simulink model "ammclib_gflib_trigonometric_s32k14x"  (Simulink 9.0)
settings: Solver=FixedStepDiscrete  StartTime=0.0  StopTime=5  FixedStep=0.001  RelTol=1e-3  EnableMultiTasking=on
InitFcn:
  | mbd_s32k_consistency_checks(bdroot(gcs));
undefined symbols (not defined in the file or in its folder): LQFP
libraries: ammclib_bam_s32k14x x70, mbd_s32k1xx_ec_toolbox x2, simulink x1
Description:
  | This model tests the AMMCLIB GFLIB TRIGONOMETRIC blocks
  | 
  | Validation:
  | - Run the model in Simulation and check the results
  | - Open Freemaster (ammclib_gflib_trigonometric_s32k14x.pmp) and compare the HW results against the Simulated ones
CloseFcn:
  | clear all;
settings Model: Creator=NXP MBDT Team  LastModifiedBy=nxf35172
settings DataIOCC: ExternalInput=off  InitialState=off  LimitDataPoints=on  SaveOutput=off  SignalLogging=off  SaveTime=off
settings OptimizationCC: DefaultParameterBehavior=Inlined  LifeSpan=1
settings DebuggingCC: SolverPrmCheckMsg=warning  InheritedTsInSrcMsg=none  SingleTaskRateTransMsg=error  IntegerOverflowMsg=none  ParameterPrecisionLossMsg=none  UnconnectedInputMsg=error  UnconnectedOutputMsg=error  UnconnectedLineMsg=error  AllowSymbolicDim=off  UnknownTsInhSupMsg=error  StateNameClashWarn=warning
settings HardwareCC: ProdLargestAtomicInteger=Long  ProdLargestAtomicFloat=Double  ProdEndianess=LittleEndian  ProdHWDeviceType=ARM Compatible->ARM Cortex
settings SFSimCC: MATLABDynamicMemAlloc=off
settings RTWCC: SystemTargetFile=mbd_s32k.tlc  MakeCommand=mbd_s32k_make_rtw COPY_MDLREF_INCLUDES=0  TemplateMakefile=mbd_s32k.tmf  Description=Model Based Design Toolbox S32K14x Code Generation Target
settings CodeAppCC: IgnoreCustomStorageClasses=off
settings STFCustomTargetCC: CombineOutputUpdateFcns=on  ERTCustomFileBanners=on  SupportContinuousTime=off  SupportNonInlinedSFcns=off  RemoveResetFunc=on  MATLABClassNameForMDSCustomization=Simulink.SoftwareTarget.ERTCustomization  GRTInterface=off  SystemTargetFile=mbd_s32k14.tlc
settings ERTTargetCC: MultiwordLength=2048  ParMdlRefBuildCompliant=off  CompOptLevelCompliant=off  ConcurrentExecutionCompliant=off  ModelStepFunctionPrototypeControlCompliant=off  CPPClassGenCompliant=off  UseToolchainInfoCompliant=off  InlinedParameterPlacement=NonHierarchical  ERTCustomFileTemplate=example_file_process.tlc  ConvertIfToSwitch=off  SuppressUnreachableDefaultCases=off

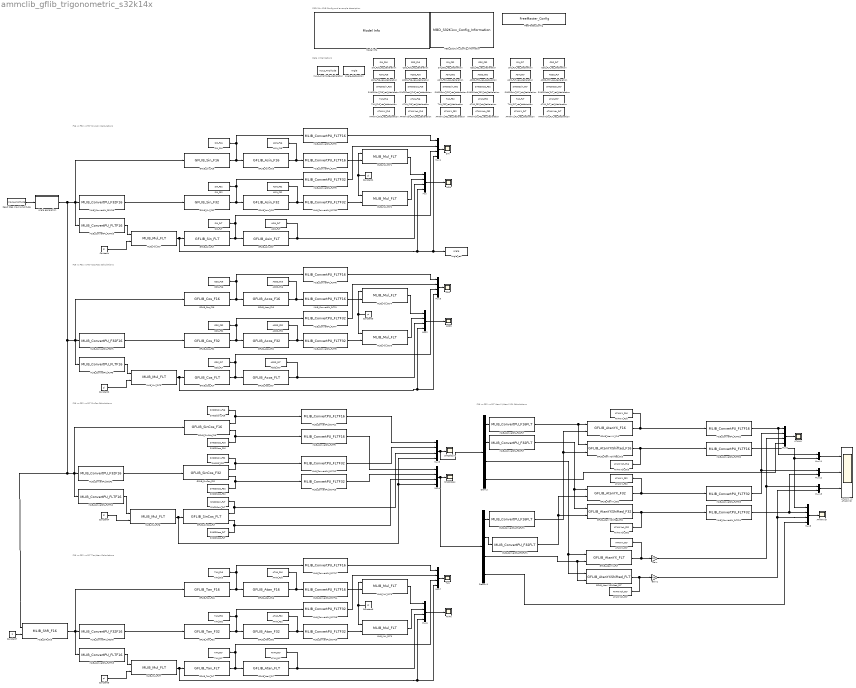
== system ammclib_gflib_trigonometric_s32k14x ==
  note: S32K14x EVB Config and example description
  note: Data Initializations
  note: F16 vs F32 vs FLT Sin/Asin Calculations
  note: F16 vs F32 vs FLT Cos/Acos Calculations
  note: F16 vs F32 vs FLT SinCos Calculations
  note: F16 vs F32 vs FLT Tan/Atan Calculations
  note: F16 vs F32 vs FLT AtanYX/AtanYXSh Calculations
  ACOS : Scope
  ACOS_F16 : DataStoreWrite  DataStoreName=ACOS_F16
  ACOS_F16_res_declaration : DataStoreMemory  Priority=2  DataStoreName=ACOS_F16  ReadBeforeWriteMsg=warning  WriteAfterWriteMsg=warning  WriteAfterReadMsg=warning  ShowAdditionalParam=off  OutDataTypeStr=int16
  ACOS_F32 : DataStoreWrite  DataStoreName=ACOS_F32
  ACOS_F32_res_declaration : DataStoreMemory  Priority=2  DataStoreName=ACOS_F32  ReadBeforeWriteMsg=warning  WriteAfterWriteMsg=warning  WriteAfterReadMsg=warning  ShowAdditionalParam=off  OutDataTypeStr=int32
  ACOS_FLT : DataStoreWrite  DataStoreName=ACOS_FLT
  ACOS_FLT_res_declaration : DataStoreMemory  Priority=2  DataStoreName=ACOS_FLT  ReadBeforeWriteMsg=warning  WriteAfterWriteMsg=warning  WriteAfterReadMsg=warning  ShowAdditionalParam=off  OutDataTypeStr=single
  ASIN : Scope
  ASIN_F16 : DataStoreWrite  DataStoreName=ASIN_F16
  ASIN_F16_res_declaration : DataStoreMemory  Priority=2  DataStoreName=ASIN_F16  ReadBeforeWriteMsg=warning  WriteAfterWriteMsg=warning  WriteAfterReadMsg=warning  ShowAdditionalParam=off  OutDataTypeStr=int16
  ASIN_F32 : DataStoreWrite  DataStoreName=ASIN_F32
  ASIN_F32_res_declaration : DataStoreMemory  Priority=2  DataStoreName=ASIN_F32  ReadBeforeWriteMsg=warning  WriteAfterWriteMsg=warning  WriteAfterReadMsg=warning  ShowAdditionalParam=off  OutDataTypeStr=int32
  ASIN_FLT : DataStoreWrite  DataStoreName=ASIN_FLT
  ASIN_FLT_res_declaration : DataStoreMemory  Priority=2  DataStoreName=ASIN_FLT  ReadBeforeWriteMsg=warning  WriteAfterWriteMsg=warning  WriteAfterReadMsg=warning  ShowAdditionalParam=off  OutDataTypeStr=single
  ATAN : Scope
  ATANXY : Scope
  ATANXYsh : Scope
  ATANYX vs ATANXYsh : Scope  NumInputPorts=3
  ATANYX_F16 : DataStoreWrite  DataStoreName=ATANYX_F16
  ATANYX_F16_res_declaration : DataStoreMemory  Priority=2  DataStoreName=ATANYX_F16  ReadBeforeWriteMsg=warning  WriteAfterWriteMsg=warning  WriteAfterReadMsg=warning  ShowAdditionalParam=off  OutDataTypeStr=int16
  ATANYX_F32 : DataStoreWrite  DataStoreName=ATANYX_F32
  ATANYX_F32_res_declaration : DataStoreMemory  Priority=2  DataStoreName=ATANYX_F32  ReadBeforeWriteMsg=warning  WriteAfterWriteMsg=warning  WriteAfterReadMsg=warning  ShowAdditionalParam=off  OutDataTypeStr=int32
  ATANYX_FLT : DataStoreWrite  DataStoreName=ATANYX_FLT
  ATANYX_FLT_res_declaration : DataStoreMemory  Priority=2  DataStoreName=ATANYX_FLT  ReadBeforeWriteMsg=warning  WriteAfterWriteMsg=warning  WriteAfterReadMsg=warning  ShowAdditionalParam=off  OutDataTypeStr=single
  ATANYXsh_F16 : DataStoreWrite  DataStoreName=ATANYXsh_F16
  ATANYXsh_F16_res_declaration : DataStoreMemory  Priority=2  DataStoreName=ATANYXsh_F16  ReadBeforeWriteMsg=warning  WriteAfterWriteMsg=warning  WriteAfterReadMsg=warning  ShowAdditionalParam=off  OutDataTypeStr=int16
  ATANYXsh_F32 : DataStoreWrite  DataStoreName=ATANYXsh_F32
  ATANYXsh_F32_res_declaration : DataStoreMemory  Priority=2  DataStoreName=ATANYXsh_F32  ReadBeforeWriteMsg=warning  WriteAfterWriteMsg=warning  WriteAfterReadMsg=warning  ShowAdditionalParam=off  OutDataTypeStr=int32
  ATANYXsh_FLT : DataStoreWrite  DataStoreName=ATANYXsh_FLT
  ATANYXsh_FLT_res_declaration : DataStoreMemory  Priority=2  DataStoreName=ATANYXsh_FLT  ReadBeforeWriteMsg=warning  WriteAfterWriteMsg=warning  WriteAfterReadMsg=warning  ShowAdditionalParam=off  OutDataTypeStr=single
  ATAN_F16 : DataStoreWrite  DataStoreName=ATAN_F16
  ATAN_F16_res_declaration : DataStoreMemory  Priority=2  DataStoreName=ATAN_F16  ReadBeforeWriteMsg=warning  WriteAfterWriteMsg=warning  WriteAfterReadMsg=warning  ShowAdditionalParam=off  OutDataTypeStr=int16
  ATAN_F32 : DataStoreWrite  DataStoreName=ATAN_F32
  ATAN_F32_res_declaration : DataStoreMemory  Priority=2  DataStoreName=ATAN_F32  ReadBeforeWriteMsg=warning  WriteAfterWriteMsg=warning  WriteAfterReadMsg=warning  ShowAdditionalParam=off  OutDataTypeStr=int32
  ATAN_FLT : DataStoreWrite  DataStoreName=ATAN_FLT
  ATAN_FLT_res_declaration : DataStoreMemory  Priority=2  DataStoreName=ATAN_FLT  ReadBeforeWriteMsg=warning  WriteAfterWriteMsg=warning  WriteAfterReadMsg=warning  ShowAdditionalParam=off  OutDataTypeStr=single
  Angle generation : Subsystem
  Angle_declaration : DataStoreMemory  Priority=1  DataStoreName=Angle  WriteAfterWriteMsg=warning  WriteAfterReadMsg=warning  ShowAdditionalParam=off  OutMin=-1  OutMax=1  OutDataTypeStr=single
  Angle_res : DataStoreWrite  DataStoreName=Angle
  COS : Scope
  COS_F16 : DataStoreWrite  DataStoreName=COS_F16
  COS_F16_res_declaration : DataStoreMemory  Priority=2  DataStoreName=COS_F16  ReadBeforeWriteMsg=warning  WriteAfterWriteMsg=warning  WriteAfterReadMsg=warning  ShowAdditionalParam=off  OutDataTypeStr=int16
  COS_F32 : DataStoreWrite  DataStoreName=COS_F32
  COS_F32_res_declaration : DataStoreMemory  Priority=2  DataStoreName=COS_F32  ReadBeforeWriteMsg=warning  WriteAfterWriteMsg=warning  WriteAfterReadMsg=warning  ShowAdditionalParam=off  OutDataTypeStr=int32
  COS_FLT : DataStoreWrite  DataStoreName=COS_FLT
  COS_FLT_res_declaration : DataStoreMemory  Priority=2  DataStoreName=COS_FLT  ReadBeforeWriteMsg=warning  WriteAfterWriteMsg=warning  WriteAfterReadMsg=warning  ShowAdditionalParam=off  OutDataTypeStr=single
  Constant{,1..6} (7 alike) : Constant  Value=pi  OutDataTypeStr=Inherit: Inherit via back propagation
  Constant7 : Constant  Value=2  OutDataTypeStr=Inherit: Inherit via back propagation
  Demux : Demux
  Demux1 : Demux
  FreeMaster_Config : mbd_s32k1xx_ec_toolbox/Utility Blocks/FreeMaster_Config  interface=LPUART1  baudrate=115200  rxd=PTC6: [LPUART1_RX | Receive]  txd=PTC7: [LPUART1_TX | Transmit]  mode=Short Interrupt  isr_prio=15  show_adv_opts=off  use_scope=on  max_scope_vars=8  use_recorder=on  max_rec_vars=8  rec_buff_size=1024  rec_timebase=0 milliseconds  comm_buffer_size_auto=on  comm_buffer_size=255  comm_rqueue_size_default=on  comm_rqueue_size=32
  GFLIB_Acos_F16 : ammclib_bam_s32k14x/GFLIB/bam_f16/GFLIB_Acos_F16
  GFLIB_Acos_F32 : ammclib_bam_s32k14x/GFLIB/bam_f32/GFLIB_Acos_F32
  GFLIB_Acos_FLT : ammclib_bam_s32k14x/GFLIB/bam_flt/GFLIB_Acos_FLT
  GFLIB_Asin_F16 : ammclib_bam_s32k14x/GFLIB/bam_f16/GFLIB_Asin_F16
  GFLIB_Asin_F32 : ammclib_bam_s32k14x/GFLIB/bam_f32/GFLIB_Asin_F32
  GFLIB_Asin_FLT : ammclib_bam_s32k14x/GFLIB/bam_flt/GFLIB_Asin_FLT
  GFLIB_AtanYXShifted_F16 : ammclib_bam_s32k14x/GFLIB/bam_f16/GFLIB_AtanYXShifted_F16  Ky=19918  Kx=28803  Ny=0  Nx=0  ThetaAdj=1820
  GFLIB_AtanYXShifted_F32 : ammclib_bam_s32k14x/GFLIB/bam_f32/GFLIB_AtanYXShifted_F32  Ky=1.305434611595101e+09  Kx=1.887749824036660e+09  Ny=0  Nx=0  ThetaAdj=1.193046470436251e+08
  GFLIB_AtanYXShifted_FLT : ammclib_bam_s32k14x/GFLIB/bam_flt/GFLIB_AtanYXShifted_FLT  Ky=0.6079089139  Kx=0.8790788409  ThetaAdj=0.1745329252
  GFLIB_AtanYX_F16 : ammclib_bam_s32k14x/GFLIB/bam_f16/GFLIB_AtanYX_F16
  GFLIB_AtanYX_F32 : ammclib_bam_s32k14x/GFLIB/bam_f32/GFLIB_AtanYX_F32
  GFLIB_AtanYX_FLT : ammclib_bam_s32k14x/GFLIB/bam_flt/GFLIB_AtanYX_FLT
  GFLIB_Atan_F16 : ammclib_bam_s32k14x/GFLIB/bam_f16/GFLIB_Atan_F16
  GFLIB_Atan_F32 : ammclib_bam_s32k14x/GFLIB/bam_f32/GFLIB_Atan_F32
  GFLIB_Atan_FLT : ammclib_bam_s32k14x/GFLIB/bam_flt/GFLIB_Atan_FLT
  GFLIB_Cos_F16 : ammclib_bam_s32k14x/GFLIB/bam_f16/GFLIB_Cos_F16
  GFLIB_Cos_F32 : ammclib_bam_s32k14x/GFLIB/bam_f32/GFLIB_Cos_F32
  GFLIB_Cos_FLT : ammclib_bam_s32k14x/GFLIB/bam_flt/GFLIB_Cos_FLT
  GFLIB_SinCos_F16 : ammclib_bam_s32k14x/GFLIB/bam_f16/GFLIB_SinCos_F16
  GFLIB_SinCos_F32 : ammclib_bam_s32k14x/GFLIB/bam_f32/GFLIB_SinCos_F32
  GFLIB_SinCos_FLT : ammclib_bam_s32k14x/GFLIB/bam_flt/GFLIB_SinCos_FLT
  GFLIB_Sin_F16 : ammclib_bam_s32k14x/GFLIB/bam_f16/GFLIB_Sin_F16
  GFLIB_Sin_F32 : ammclib_bam_s32k14x/GFLIB/bam_f32/GFLIB_Sin_F32
  GFLIB_Sin_FLT : ammclib_bam_s32k14x/GFLIB/bam_flt/GFLIB_Sin_FLT
  GFLIB_Tan_F16 : ammclib_bam_s32k14x/GFLIB/bam_f16/GFLIB_Tan_F16
  GFLIB_Tan_F32 : ammclib_bam_s32k14x/GFLIB/bam_f32/GFLIB_Tan_F32
  GFLIB_Tan_FLT : ammclib_bam_s32k14x/GFLIB/bam_flt/GFLIB_Tan_FLT
  Gain : Gain  Gain=1/pi
  Gain1 : Gain  Gain=1/pi
  Input_Amplitude_declaration : DataStoreMemory  Priority=1  DataStoreName=Input_Amplitude  WriteAfterWriteMsg=warning  WriteAfterReadMsg=warning  InitialValue=3.14  ShowAdditionalParam=off  OutMin=-pi  OutMax=pi  OutDataTypeStr=single
  MBD_S32K14x_Config_Information : mbd_s32k1xx_ec_toolbox/MBD_S32K1xx_Config_Information  Priority=0  mbdt_ver=0  disp_str=|  config_params=[]  mcu_target_name=S32K144  mcu_target_package=100-LQFP  mcu_target_sram_size=64KB  mcu_system_clock_freq=80  mcu_xtal_freq=External 8  mcu_steptick_timer=LPIT Channel 0  mcu_steptick_prio=15  ds_import_enable=on  target_compiler=GCC  target_memory=FLASH  gcc_target_compile_opts=-mcpu=cortex-m4 -mthumb -mfloat-abi=hard -mfpu=fpv4-sp-d16 -O1 -g -gstrict-dwarf  gcc_target_assemble_opts=-mcpu=cortex-m4 -mthumb -mfloat-abi=hard -mfpu=fpv4-sp-d16 -g  gcc_target_link_opts=-mcpu=cortex-m4 -mthumb -mfloat-abi=hard -mfpu=fpv4-sp-d16  gcc_target_default_lcf=on  gcc_target_user_lcf=S32K144_64_flash.ld  ghs_target_compile_opts=-cpu=cortexm4f -thumb -DARM_MATH_CM4 -fpu=vfpv4_d16 -fsingle -Ogeneral -Wundef -Wimplicit-int -Wshadow -Wtrigraphs --no_commons --gnu_asm -gnu99 -gdwarf-2 -G  ghs_target_assemble_opts=-cpu=cortexm4f -fpu=vfpv4_d16  ghs_target_link_opts=-cpu=cortexm4f -thumb -fpu=vfpv4_d16  ghs_target_default_lcf=off  ghs_target_user_lcf=S32K144_64_flash.ld  iar_target_compile_opts=--cpu=Cortex-M4F --thumb --fpu=VFPv4_sp -Ol -e --debug --dlib_config normal  iar_target_assemble_opts=--cpu Cortex-M4F --thumb --fpu VFPv4_sp  iar_target_link_opts=--no_exceptions --vfe --inline  iar_target_default_lcf=off  iar_target_user_lcf=S32K144_64_flash.icf  pil_download_enable=off  rbl_download_enable=on  rbl_start_delay=5000000  rbl_download_interface=OpenSDA  rbl_restart_request=off  rbl_com_port=Custom  rbl_com_port_custom=COM1  pil_download_rate=57600  pil_opensda_drive=Custom  pil_opensda_drive_custom=D  pil_uart_instance=1  pil_uart_rx=PTC6: [LPUART1_RX | Receive]  pil_uart_tx=PTC7: [LPUART1_TX | Transmit]  FTM_PWM_PcrCheckEnDis=on  FTM_Input_Edge_Inputs_PcrCheckEnDis=on  FTM_Dual_Edge_Inputs_PcrCheckEnDis=on  FTM_Quadrature_Inputs_PcrCheckEnDis=on  FTM_Hall_Sensor_Inputs_PcrCheckEnDis=on  LPTMR_PcrCheckEnDis=on  PIT_PcrCheckEnDis=on  RTC_PcrCheckEnDis=on  FlexCAN_PcrCheckEnDis=on  LIN_PcrCheckEnDis=on  FlexIO_PcrCheckEnDis=on  LPI2C_PcrCheckEnDis=on  LPSPI_PcrCheckEnDis=on  LPUART_PcrCheckEnDis=on  CMP_PcrCheckEnDis=on  GPIO_OutputPcrCheckEnDis=on  GPIO_InputPcrCheckEnDis=on  SBC_PcrCheckEnDis=on  AMMCLIB_PcrCheckEnDis=on  FM_PcrCheckEnDis=on  Profile_PcrCheckEnDis=on  ConfigParams_PcrCheckEnDis=on  ModelRef_PcrCheckEnDis=on  PDB0_PcrCheckEnDis=on  CSEc_PcrCheckEnDis=on  eDMA_PcrCheckEnDis=on  ADC_PcrCheckEnDis=on  WDOG_PcrCheckEnDis=on
      | Target : S32K142-16KB_SRAM
      | Package : 100-pin
      | System clock : 80 MHz
      | XTAL clock : External 8 MHz
      | Compiler : GCC
      | Target Type : FLASH
      | Download Code after build : (OpenSDA: E)
      | Step Tick Interrupt Priority : 15
  MLIB_ConvertPU_F16FLT : ammclib_bam_s32k14x/MLIB/bam_f16/MLIB_ConvertPU_F16FLT
  MLIB_ConvertPU_F16FLT1 : ammclib_bam_s32k14x/MLIB/bam_f16/MLIB_ConvertPU_F16FLT
  MLIB_ConvertPU_F32F{1..3,16} (4 alike) : ammclib_bam_s32k14x/MLIB/bam_f32/MLIB_ConvertPU_F32F16
  MLIB_ConvertPU_F32FLT : ammclib_bam_s32k14x/MLIB/bam_f32/MLIB_ConvertPU_F32FLT
  MLIB_ConvertPU_F32FLT1 : ammclib_bam_s32k14x/MLIB/bam_f32/MLIB_ConvertPU_F32FLT
  MLIB_ConvertPU_FLTF{1..2,4..6,9..11,14..17,20,22} (14 alike) : ammclib_bam_s32k14x/MLIB/bam_flt/MLIB_ConvertPU_FLTF16
  MLIB_ConvertPU_FLTF{3,7..8,12..13,18..19,23..24,32} (10 alike) : ammclib_bam_s32k14x/MLIB/bam_flt/MLIB_ConvertPU_FLTF32
  MLIB_Mul_FLT{,1..9} (10 alike) : ammclib_bam_s32k14x/MLIB/bam_flt/MLIB_Mul_FLT
  MLIB_ShR_F16 : ammclib_bam_s32k14x/MLIB/bam_f16/MLIB_ShR_F16
  Model Info : simulink/Model-Wide Utilities/Model Info  Frame=off  DisplayStringWithTags=|  HorizontalTextAlignment=Left  LeftAlignmentValue=0.02
      | Model Name: %<ModelName>
      | 
      | Description: %<Description>
  Mux{,1..9} (10 alike) : Mux
  Mux11 : Mux  Inputs=2
  Mux12 : Mux  Inputs=2
  Mux13 : Mux  Inputs=2
  Read Step Input Amplitude : DataStoreRead  DataStoreName=Input_Amplitude
  SIN : Scope
  SINCOS_F32 : DataStoreWrite  DataStoreName=SINCOSsin_F32
  SINCOScos : Scope
  SINCOScos_F16 : DataStoreWrite  DataStoreName=SINCOScos_F16
  SINCOScos_F16_res_declaration : DataStoreMemory  Priority=2  DataStoreName=SINCOScos_F16  ReadBeforeWriteMsg=warning  WriteAfterWriteMsg=warning  WriteAfterReadMsg=warning  ShowAdditionalParam=off  OutDataTypeStr=int16
  SINCOScos_F32 : DataStoreWrite  DataStoreName=SINCOScos_F32
  SINCOScos_F32_res_declaration : DataStoreMemory  Priority=2  DataStoreName=SINCOScos_F32  ReadBeforeWriteMsg=warning  WriteAfterWriteMsg=warning  WriteAfterReadMsg=warning  ShowAdditionalParam=off  OutDataTypeStr=int32
  SINCOScos_FLT : DataStoreWrite  DataStoreName=SINCOScos_FLT
  SINCOScos_FLT_res_declaration : DataStoreMemory  Priority=2  DataStoreName=SINCOScos_FLT  ReadBeforeWriteMsg=warning  WriteAfterWriteMsg=warning  WriteAfterReadMsg=warning  ShowAdditionalParam=off  OutDataTypeStr=single
  SINCOSsin : Scope
  SINCOSsin_F16 : DataStoreWrite  DataStoreName=SINCOSsin_F16
  SINCOSsin_F16_res_declaration : DataStoreMemory  Priority=2  DataStoreName=SINCOSsin_F16  ReadBeforeWriteMsg=warning  WriteAfterWriteMsg=warning  WriteAfterReadMsg=warning  ShowAdditionalParam=off  OutDataTypeStr=int16
  SINCOSsin_F32_res_declaration : DataStoreMemory  Priority=2  DataStoreName=SINCOSsin_F32  ReadBeforeWriteMsg=warning  WriteAfterWriteMsg=warning  WriteAfterReadMsg=warning  ShowAdditionalParam=off  OutDataTypeStr=int32
  SINCOSsin_FLT : DataStoreWrite  DataStoreName=SINCOSsin_FLT
  SINCOSsin_FLT_res_declaration : DataStoreMemory  Priority=2  DataStoreName=SINCOSsin_FLT  ReadBeforeWriteMsg=warning  WriteAfterWriteMsg=warning  WriteAfterReadMsg=warning  ShowAdditionalParam=off  OutDataTypeStr=single
  SIN_F16 : DataStoreWrite  DataStoreName=SIN_F16
  SIN_F16_res_declaration : DataStoreMemory  Priority=2  DataStoreName=SIN_F16  ReadBeforeWriteMsg=warning  WriteAfterWriteMsg=warning  WriteAfterReadMsg=warning  ShowAdditionalParam=off  OutDataTypeStr=int16
  SIN_F32 : DataStoreWrite  DataStoreName=SIN_F32
  SIN_F32_res_declaration : DataStoreMemory  Priority=2  DataStoreName=SIN_F32  ReadBeforeWriteMsg=warning  WriteAfterWriteMsg=warning  WriteAfterReadMsg=warning  ShowAdditionalParam=off  OutDataTypeStr=int32
  SIN_FLT : DataStoreWrite  DataStoreName=SIN_FLT
  SIN_FLT_res_declaration : DataStoreMemory  Priority=2  DataStoreName=SIN_FLT  ReadBeforeWriteMsg=warning  WriteAfterWriteMsg=warning  WriteAfterReadMsg=warning  ShowAdditionalParam=off  OutDataTypeStr=single
  TAN : Scope
  TAN_F16 : DataStoreWrite  DataStoreName=TAN_F16
  TAN_F16_res_declaration : DataStoreMemory  Priority=2  DataStoreName=TAN_F16  ReadBeforeWriteMsg=warning  WriteAfterWriteMsg=warning  WriteAfterReadMsg=warning  ShowAdditionalParam=off  OutDataTypeStr=int16
  TAN_F32 : DataStoreWrite  DataStoreName=TAN_F32
  TAN_F32_res_declaration : DataStoreMemory  Priority=2  DataStoreName=TAN_F32  ReadBeforeWriteMsg=warning  WriteAfterWriteMsg=warning  WriteAfterReadMsg=warning  ShowAdditionalParam=off  OutDataTypeStr=int32
  TAN_FLT : DataStoreWrite  DataStoreName=TAN_FLT
  TAN_FLT_res_declaration : DataStoreMemory  Priority=2  DataStoreName=TAN_FLT  ReadBeforeWriteMsg=warning  WriteAfterWriteMsg=warning  WriteAfterReadMsg=warning  ShowAdditionalParam=off  OutDataTypeStr=single
  wires:
  GFLIB_Sin_F16/1 -> MLIB_ConvertPU_FLTF2/1, SIN_F16/1, GFLIB_Asin_F16/1
  MLIB_ConvertPU_F32F16/1 -> GFLIB_Sin_F32/1
  GFLIB_Sin_F32/1 -> MLIB_ConvertPU_FLTF3/1, SIN_F32/1, GFLIB_Asin_F32/1
  GFLIB_Sin_FLT/1 -> Mux1/3, SIN_FLT/1, GFLIB_Asin_FLT/1  "SIN_FLT"
  MLIB_ConvertPU_FLTF16/1 -> MLIB_Mul_FLT/1
  Constant/1 -> MLIB_Mul_FLT/2
  MLIB_Mul_FLT/1 -> Mux/4, Angle_res/1, Mux1/4, GFLIB_Sin_FLT/1  "Angle[rad]"
  Mux/1 -> ASIN/1
  GFLIB_Asin_F16/1 -> ASIN_F16/1, MLIB_ConvertPU_FLTF1/1
  GFLIB_Asin_FLT/1 -> ASIN_FLT/1, Mux/3  "ASIN_FLT"
  GFLIB_Asin_F32/1 -> ASIN_F32/1, MLIB_ConvertPU_FLTF32/1
  MLIB_ConvertPU_FLTF1/1 -> MLIB_Mul_FLT1/2
  Constant1/1 -> MLIB_Mul_FLT1/1, MLIB_Mul_FLT2/1
  MLIB_Mul_FLT1/1 -> Mux/1  "ASIN_F16"
  MLIB_ConvertPU_FLTF32/1 -> MLIB_Mul_FLT2/2
  MLIB_Mul_FLT2/1 -> Mux/2  "ASIN_F32"
  Mux1/1 -> SIN/1
  MLIB_ConvertPU_FLTF2/1 -> Mux1/1  "SIN_F16"
  MLIB_ConvertPU_FLTF3/1 -> Mux1/2  "SIN_F32"
  Read Step Input Amplitude/1 -> Angle generation/1("Amplitude ")
  GFLIB_Cos_F16/1 -> GFLIB_Acos_F16/1, MLIB_ConvertPU_FLTF6/1, COS_F16/1
  MLIB_ConvertPU_F32F1/1 -> GFLIB_Cos_F32/1
  GFLIB_Cos_F32/1 -> GFLIB_Acos_F32/1, MLIB_ConvertPU_FLTF7/1, COS_F32/1
  GFLIB_Cos_FLT/1 -> GFLIB_Acos_FLT/1, Mux3/3, COS_FLT/1  "COS_FLT"
  MLIB_ConvertPU_FLTF5/1 -> MLIB_Mul_FLT3/1
  Constant2/1 -> MLIB_Mul_FLT3/2
  MLIB_Mul_FLT3/1 -> GFLIB_Cos_FLT/1, Mux2/4, Mux3/4  "Angle[rad]"
  Mux2/1 -> ACOS/1
  GFLIB_Acos_F16/1 -> ACOS_F16/1, MLIB_ConvertPU_FLTF4/1
  GFLIB_Acos_FLT/1 -> ACOS_FLT/1, Mux2/3  "ACOS_FLT"
  GFLIB_Acos_F32/1 -> ACOS_F32/1, MLIB_ConvertPU_FLTF8/1
  MLIB_ConvertPU_FLTF4/1 -> MLIB_Mul_FLT4/2
  Constant3/1 -> MLIB_Mul_FLT4/1, MLIB_Mul_FLT5/1
  MLIB_Mul_FLT4/1 -> Mux2/1  "ACOS_F16"
  MLIB_ConvertPU_FLTF8/1 -> MLIB_Mul_FLT5/2
  MLIB_Mul_FLT5/1 -> Mux2/2  "ACOS_F32"
  Mux3/1 -> COS/1
  MLIB_ConvertPU_FLTF6/1 -> Mux3/1  "COS_F16"
  MLIB_ConvertPU_FLTF7/1 -> Mux3/2  "COS_F32"
  GFLIB_SinCos_F16/1 -> SINCOSsin_F16/1, MLIB_ConvertPU_FLTF11/1
  MLIB_ConvertPU_F32F2/1 -> GFLIB_SinCos_F32/1
  GFLIB_SinCos_F32/1 -> MLIB_ConvertPU_FLTF12/1, SINCOS_F32/1
  GFLIB_SinCos_FLT/1 -> Mux5/3, SINCOSsin_FLT/1  "SINCOSsin_FLT"
  MLIB_ConvertPU_FLTF10/1 -> MLIB_Mul_FLT6/1
  Constant4/1 -> MLIB_Mul_FLT6/2
  Mux5/1 -> Demux/1, SINCOSsin/1
  MLIB_ConvertPU_FLTF11/1 -> Mux5/1  "SINCOSsin_F16"
  MLIB_ConvertPU_FLTF12/1 -> Mux5/2  "SINCOSsin_F32"
  GFLIB_SinCos_F16/2 -> SINCOScos_F16/1, MLIB_ConvertPU_FLTF9/1
  GFLIB_SinCos_F32/2 -> MLIB_ConvertPU_FLTF13/1, SINCOScos_F32/1
  GFLIB_SinCos_FLT/2 -> Mux4/3, SINCOScos_FLT/1  "SINCOScos_FLT"
  Mux4/1 -> Demux1/1, SINCOScos/1
  MLIB_ConvertPU_FLTF9/1 -> Mux4/1  "SINCOScos_F16"
  MLIB_ConvertPU_FLTF13/1 -> Mux4/2  "SINCOScos-F32"
  GFLIB_Tan_F16/1 -> GFLIB_Atan_F16/1, MLIB_ConvertPU_FLTF17/1, TAN_F16/1
  MLIB_ConvertPU_F32F3/1 -> GFLIB_Tan_F32/1
  GFLIB_Tan_F32/1 -> GFLIB_Atan_F32/1, MLIB_ConvertPU_FLTF18/1, TAN_F32/1
  GFLIB_Tan_FLT/1 -> GFLIB_Atan_FLT/1, Mux7/3, TAN_FLT/1  "TAN_FLT"
  MLIB_ConvertPU_FLTF15/1 -> MLIB_Mul_FLT7/1
  Constant5/1 -> MLIB_Mul_FLT7/2
  MLIB_Mul_FLT7/1 -> GFLIB_Tan_FLT/1, Mux6/4, Mux7/4  "Angle[rad]"
  Mux6/1 -> ATAN/1
  GFLIB_Atan_F16/1 -> ATAN_F16/1, MLIB_ConvertPU_FLTF14/1
  GFLIB_Atan_FLT/1 -> ATAN_FLT/1, Mux6/3  "ATAN_FLT"
  GFLIB_Atan_F32/1 -> ATAN_F32/1, MLIB_ConvertPU_FLTF19/1
  MLIB_ConvertPU_FLTF14/1 -> MLIB_Mul_FLT8/2
  Constant6/1 -> MLIB_Mul_FLT8/1, MLIB_Mul_FLT9/1
  MLIB_Mul_FLT8/1 -> Mux6/1  "ATAN_F16"
  MLIB_ConvertPU_FLTF19/1 -> MLIB_Mul_FLT9/2
  MLIB_Mul_FLT9/1 -> Mux6/2  "ATAN_F32"
  Mux7/1 -> TAN/1
  MLIB_ConvertPU_FLTF17/1 -> Mux7/1  "TAN_F16"
  MLIB_ConvertPU_FLTF18/1 -> Mux7/2  "TAN_F32"
  MLIB_ShR_F16/1 -> GFLIB_Tan_F16/1, MLIB_ConvertPU_F32F3/1, MLIB_ConvertPU_FLTF15/1
  Constant7/1 -> MLIB_ShR_F16/2
  GFLIB_AtanYX_F16/1 -> ATANYX_F16/1, MLIB_ConvertPU_FLTF22/1
  GFLIB_AtanYX_F32/1 -> ATANYX_F32/1, MLIB_ConvertPU_FLTF23/1
  GFLIB_AtanYX_FLT/1 -> Gain/1, ATANYX_FLT/1  "ATANYX_FLT"
  MLIB_Mul_FLT6/1 -> GFLIB_SinCos_FLT/1, Mux4/4, Mux5/4  "Angle[rad]"
  Mux8/1 -> ATANXYsh/1
  GFLIB_AtanYXShifted_F16/1 -> ATANYXsh_F16/1, MLIB_ConvertPU_FLTF20/1
  MLIB_ConvertPU_FLTF20/1 -> Mux11/2, Mux8/1  "ATANsh_F16"
  MLIB_ConvertPU_FLTF24/1 -> Mux12/2, Mux8/2  "ATANsh_F32"
  Mux9/1 -> ATANXY/1
  MLIB_ConvertPU_FLTF22/1 -> Mux11/1, Mux9/1  "ATANYX_F16"
  MLIB_ConvertPU_FLTF23/1 -> Mux12/1, Mux9/2  "ATANYX_F32"
  Angle generation/1(Angle) -> MLIB_ShR_F16/1, MLIB_ConvertPU_FLTF10/1, MLIB_ConvertPU_F32F2/1, GFLIB_SinCos_F16/1, GFLIB_Cos_F16/1, MLIB_ConvertPU_F32F1/1, MLIB_ConvertPU_FLTF5/1, GFLIB_Sin_F16/1, MLIB_ConvertPU_F32F16/1, MLIB_ConvertPU_FLTF16/1
  GFLIB_AtanYXShifted_F32/1 -> ATANYXsh_F32/1, MLIB_ConvertPU_FLTF24/1
  GFLIB_AtanYXShifted_FLT/1 -> Gain1/1, ATANYXsh_FLT/1
  Demux/1 -> MLIB_ConvertPU_F16FLT/1
  Demux/2 -> MLIB_ConvertPU_F32FLT/1
  Demux/3 -> GFLIB_AtanYX_FLT/1, GFLIB_AtanYXShifted_FLT/1
  Demux1/1 -> MLIB_ConvertPU_F16FLT1/1
  Demux1/2 -> MLIB_ConvertPU_F32FLT1/1
  Demux/4 -> Mux9/4
  Demux1/4 -> Mux8/4
  MLIB_ConvertPU_F16FLT/1 -> GFLIB_AtanYXShifted_F16/1, GFLIB_AtanYX_F16/1
  MLIB_ConvertPU_F32FLT/1 -> GFLIB_AtanYX_F32/1, GFLIB_AtanYXShifted_F32/1
  MLIB_ConvertPU_F16FLT1/1 -> GFLIB_AtanYXShifted_F16/2, GFLIB_AtanYX_F16/2
  MLIB_ConvertPU_F32FLT1/1 -> GFLIB_AtanYX_F32/2, GFLIB_AtanYXShifted_F32/2
  Demux1/3 -> GFLIB_AtanYX_FLT/2, GFLIB_AtanYXShifted_FLT/2
  Gain/1 -> Mux13/1, Mux9/3  "ATANYX_FLT"
  Gain1/1 -> Mux8/3, Mux13/2  "ATANsh_FLT"
  Mux11/1 -> ATANYX vs ATANXYsh/1
  Mux12/1 -> ATANYX vs ATANXYsh/2
  Mux13/1 -> ATANYX vs ATANXYsh/3

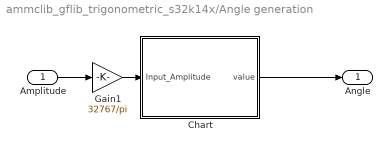
== system ammclib_gflib_trigonometric_s32k14x/Angle generation ==
  "Amplitude " : Inport
  Chart : Stateflow chart  TreatAsAtomicUnit=on
  Gain1 : Gain  Gain=32767/pi  OutDataTypeStr=Inherit: Inherit via back propagation
  Angle : Outport
  wires:
  Chart/1(value) -> Angle/1
  "Amplitude "/1 -> Gain1/1
  Gain1/1 -> Chart/1(Input_Amplitude)

== stateflow chart Angle generation/Chart ==
  settings: executeAtInitialization=1
  state A
    du:
    cntr=cntr+25;
    value=cntr;
    ex:
    cntr = -Input_Amplitude;
  (default) -> A : {cntr=0;}
  A -> A : [cntr >= Input_Amplitude]
  data: cntr local int16 =0; value output int16; Input_Amplitude input int16
